simulink library "FaultInsertionUnit"  (Simulink 8.0)
settings: Solver=ode45  StartTime=0.0  StopTime=10.0  RelTol=1e-3
undefined symbols (not defined in the file): Ts
libraries: simulink x16
(part 1 of 2)
settings Model: Creator=jroth  LastModifiedBy=jroth

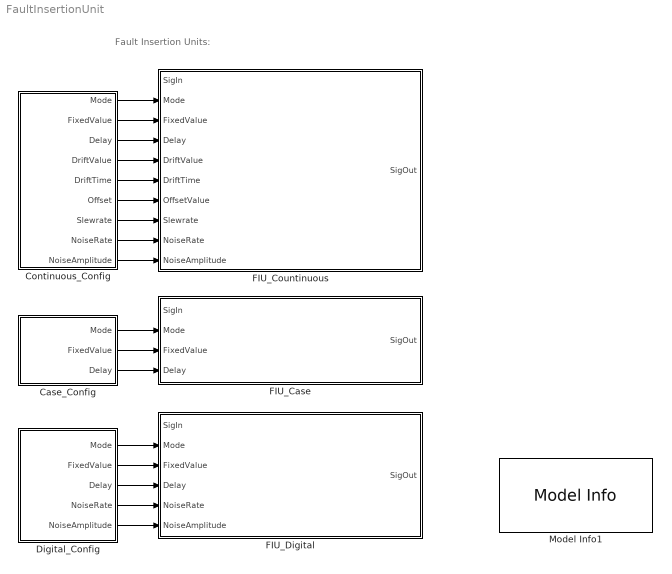
== system FaultInsertionUnit ==
  note: Fault Insertion Units:
  Case_Config : Subsystem
  Continuous_Config : Subsystem
  Digital_Config : Subsystem
  FIU_Case : Subsystem
  FIU_Countinuous : Subsystem
  FIU_Digital : Subsystem
  Model Info1 : simulink/Model-Wide Utilities/Model Info  InitialBlockCM=None  BlockCM=None  Frame=on  DisplayStringWithTags=|  HorizontalTextAlignment=Center  LeftAlignmentValue=0.5  SourceBlockDiagram=FaultInsertionUnit  TagMaxNumber=20
      | Version:
      | %<Creator>
      | %<ModifiedDate>
      | %<ModelVersion>
  wires:
  Case_Config/1(Mode) -> FIU_Case/2(Mode)
  Case_Config/2(FixedValue) -> FIU_Case/3(FixedValue)
  Case_Config/3(Delay) -> FIU_Case/4(Delay)
  Digital_Config/1(Mode) -> FIU_Digital/2(Mode)
  Digital_Config/2(FixedValue) -> FIU_Digital/3(FixedValue)
  Digital_Config/3(Delay) -> FIU_Digital/4(Delay)
  Digital_Config/4(NoiseRate) -> FIU_Digital/5(NoiseRate)
  Digital_Config/5(NoiseAmplitude) -> FIU_Digital/6(NoiseAmplitude)
  Continuous_Config/9(NoiseAmplitude) -> FIU_Countinuous/10(NoiseAmplitude)
  Continuous_Config/8(NoiseRate) -> FIU_Countinuous/9(NoiseRate)
  Continuous_Config/7(Slewrate) -> FIU_Countinuous/8(Slewrate)
  Continuous_Config/2(FixedValue) -> FIU_Countinuous/3(FixedValue)
  Continuous_Config/1(Mode) -> FIU_Countinuous/2(Mode)
  Continuous_Config/3(Delay) -> FIU_Countinuous/4(Delay)
  Continuous_Config/4(DriftValue) -> FIU_Countinuous/5(DriftValue)
  Continuous_Config/5(DriftTime) -> FIU_Countinuous/6(DriftTime)
  Continuous_Config/6(Offset) -> FIU_Countinuous/7(OffsetValue)

== system FaultInsertionUnit/Case_Config ==
  Auto Mode Selection : Subsystem
  Set Delay : Constant  Value=0
  Set FixedValue : Constant  Value=0
  Set Freeze : Constant  Value=0
  Mode : Outport
  FixedValue : Outport  Port=2
  Delay : Outport  Port=3
  wires:
  Set Delay/1 -> Delay/1, Auto Mode Selection/3(Check Delay)
  Set FixedValue/1 -> Auto Mode Selection/1(Check FixedValue), FixedValue/1
  Auto Mode Selection/1(Out1) -> Mode/1
  Set Freeze/1 -> Auto Mode Selection/2(Check Freeze)

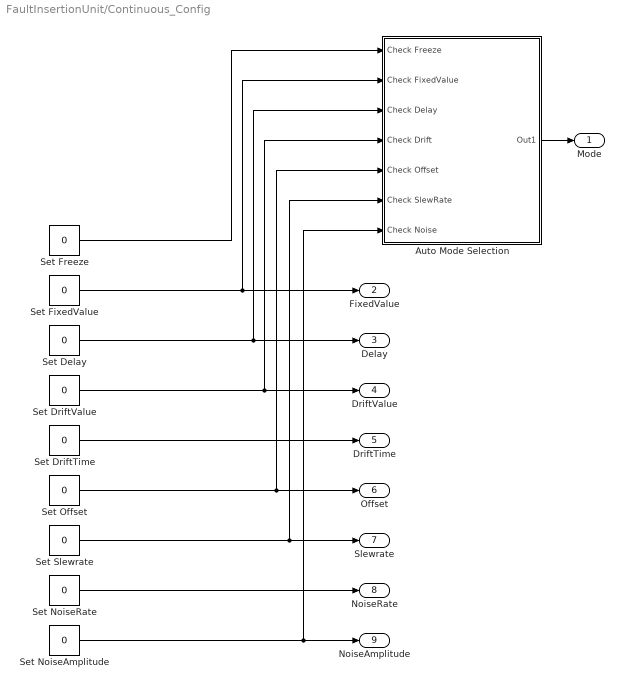
== system FaultInsertionUnit/Continuous_Config ==
  Auto Mode Selection : Subsystem
  Set Delay : Constant  Value=0
  Set DriftTime : Constant  Value=0
  Set DriftValue : Constant  Value=0
  Set FixedValue : Constant  Value=0
  Set Freeze : Constant  Value=0
  Set NoiseAmplitude : Constant  Value=0
  Set NoiseRate : Constant  Value=0
  Set Offset : Constant  Value=0
  Set Slewrate : Constant  Value=0
  Mode : Outport
  FixedValue : Outport  Port=2
  Delay : Outport  Port=3
  DriftValue : Outport  Port=4
  DriftTime : Outport  Port=5
  Offset : Outport  Port=6
  Slewrate : Outport  Port=7
  NoiseRate : Outport  Port=8
  NoiseAmplitude : Outport  Port=9
  wires:
  Set NoiseRate/1 -> NoiseRate/1
  Set Delay/1 -> Auto Mode Selection/3(Check Delay), Delay/1
  Set Offset/1 -> Auto Mode Selection/5(Check Offset), Offset/1
  Set FixedValue/1 -> Auto Mode Selection/2(Check FixedValue), FixedValue/1
  Set NoiseAmplitude/1 -> Auto Mode Selection/7(Check Noise), NoiseAmplitude/1
  Set Slewrate/1 -> Auto Mode Selection/6(Check SlewRate), Slewrate/1
  Auto Mode Selection/1(Out1) -> Mode/1
  Set DriftValue/1 -> Auto Mode Selection/4(Check Drift), DriftValue/1
  Set DriftTime/1 -> DriftTime/1
  Set Freeze/1 -> Auto Mode Selection/1(Check Freeze)

== system FaultInsertionUnit/Digital_Config ==
  Auto Mode Selection : Subsystem
  Set Delay : Constant  Value=0
  Set FixedValue : Constant  Value=0
  Set Freeze : Constant  Value=0
  Set Negate : Constant  Value=0
  Set NoiseAmplitude : Constant  Value=0
  Set NoiseRate : Constant  Value=0
  Mode : Outport
  FixedValue : Outport  Port=2
  Delay : Outport  Port=3
  NoiseRate : Outport  Port=4
  NoiseAmplitude : Outport  Port=5
  wires:
  Set NoiseRate/1 -> NoiseRate/1
  Set Delay/1 -> Auto Mode Selection/4(Check Delay), Delay/1
  Set Negate/1 -> Auto Mode Selection/2(Check Negate)
  Set FixedValue/1 -> Auto Mode Selection/1(Check FixedValue), FixedValue/1
  Set NoiseAmplitude/1 -> Auto Mode Selection/5(Check Noise), NoiseAmplitude/1
  Auto Mode Selection/1(Out1) -> Mode/1
  Set Freeze/1 -> Auto Mode Selection/3(Check Freeze)

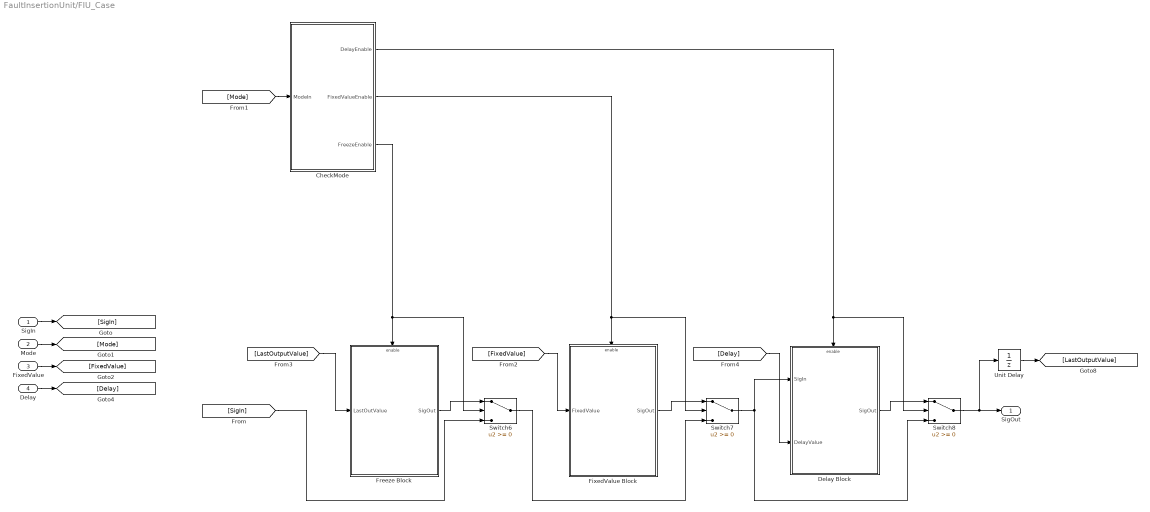
== system FaultInsertionUnit/FIU_Case ==
  SigIn : Inport
  Mode : Inport  Port=2
  FixedValue : Inport  Port=3
  Delay : Inport  Port=4
  CheckMode : Subsystem
  Delay Block : Subsystem
  FixedValue Block : Subsystem  TreatAsAtomicUnit=on
  Freeze Block : Subsystem  TreatAsAtomicUnit=on
  Switch6 : Switch
  Switch7 : Switch
  Switch8 : Switch
  Unit Delay : UnitDelay  SampleTime=-1
  SigOut : Outport
  wires:
  [FixedValue] -> FixedValue Block/1(FixedValue)
  Delay Block/1(SigOut) -> Switch8/1
  Switch7/1 -> Delay Block/1(SigIn), Switch8/3
  [Delay] -> Delay Block/2(DelayValue)
  [SigIn] -> Switch6/3
  CheckMode/3(FreezeEnable) -> Switch6/2, Freeze Block/Enable
  Switch6/1 -> Switch7/3
  CheckMode/2(FixedValueEnable) -> Switch7/2, FixedValue Block/Enable
  CheckMode/1(DelayEnable) -> Switch8/2, Delay Block/Enable
  FixedValue Block/1(SigOut) -> Switch7/1
  Freeze Block/1(SigOut) -> Switch6/1
  SigIn/1 -> [SigIn]
  Mode/1 -> [Mode]
  FixedValue/1 -> [FixedValue]
  Delay/1 -> [Delay]
  [Mode] -> CheckMode/1(ModeIn)
  Switch8/1 -> Unit Delay/1, SigOut/1
  [LastOutputValue] -> Freeze Block/1(LastOutValue)
  Unit Delay/1 -> [LastOutputValue]

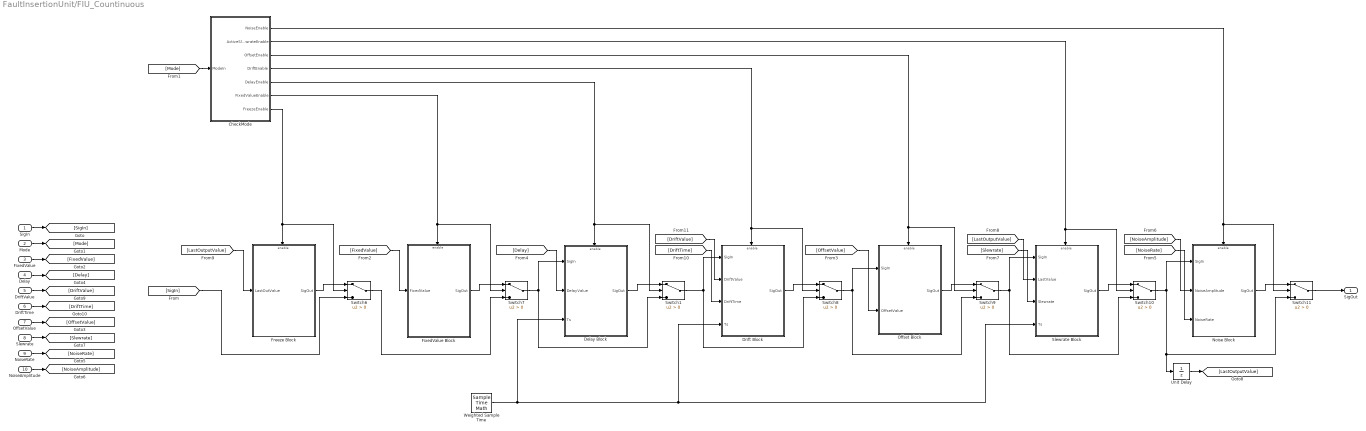
== system FaultInsertionUnit/FIU_Countinuous ==
  SigIn : Inport
  Mode : Inport  Port=2
  FixedValue : Inport  Port=3
  Delay : Inport  Port=4
  DriftValue : Inport  Port=5
  DriftTime : Inport  Port=6
  OffsetValue : Inport  Port=7
  Slewrate : Inport  Port=8
  NoiseRate : Inport  Port=9
  NoiseAmplitude : Inport  Port=10
  CheckMode : Subsystem
  Delay Block : Subsystem
  Drift Block : Subsystem  TreatAsAtomicUnit=on
  FixedValue Block : Subsystem  TreatAsAtomicUnit=on
  Freeze Block : Subsystem  TreatAsAtomicUnit=on
      mask Display: image(imread('freeze.jpg'))
  Noise Block : Subsystem
  Offset Block : Subsystem
  Slewrate Block : Subsystem
  Switch{1,6..11} (7 alike) : Switch  Criteria=u2 > Threshold
  Unit Delay : UnitDelay  SampleTime=-1
  Weighted Sample Time : SampleTimeMath  TsampMathOp=Ts Only
  SigOut : Outport
  wires:
  [FixedValue] -> FixedValue Block/1(FixedValue)
  Slewrate Block/1(SigOut) -> Switch10/1
  [Slewrate] -> Slewrate Block/3(Slewrate)
  Offset Block/1(SigOut) -> Switch9/1
  Switch9/1 -> Slewrate Block/1(SigIn), Switch10/3
  [NoiseRate] -> Noise Block/3(NoiseRate)
  Switch7/1 -> Switch1/3, Delay Block/1(SigIn)
  [NoiseAmplitude] -> Noise Block/2(NoiseAmplitude)
  Switch10/1 -> Unit Delay/1, Switch11/3, Noise Block/1(SigIn)
  [Delay] -> Delay Block/2(DelayValue)
  Noise Block/1(SigOut) -> Switch11/1
  [LastOutputValue] -> Slewrate Block/2(LastValue)
  [OffsetValue] -> Offset Block/2(OffsetValue)
  Switch8/1 -> Switch9/3, Offset Block/1(SigIn)
  [SigIn] -> Switch6/3
  CheckMode/7(FreezeEnable) -> Switch6/2, Freeze Block/Enable
  Switch6/1 -> Switch7/3
  CheckMode/6(FixedValueEnable) -> Switch7/2, FixedValue Block/Enable
  CheckMode/2(ActiveSlewrateEnable) -> Switch10/2, Slewrate Block/Enable
  CheckMode/1(NoiseEnable) -> Switch11/2, Noise Block/Enable
  FixedValue Block/1(SigOut) -> Switch7/1
  Freeze Block/1(SigOut) -> Switch6/1
  SigIn/1 -> [SigIn]
  Mode/1 -> [Mode]
  FixedValue/1 -> [FixedValue]
  OffsetValue/1 -> [OffsetValue]
  Delay/1 -> [Delay]
  NoiseRate/1 -> [NoiseRate]
  NoiseAmplitude/1 -> [NoiseAmplitude]
  Slewrate/1 -> [Slewrate]
  Unit Delay/1 -> [LastOutputValue]
  [Mode] -> CheckMode/1(ModeIn)
  Switch11/1 -> SigOut/1
  [LastOutputValue] -> Freeze Block/1(LastOutValue)
  CheckMode/3(OffsetEnable) -> Offset Block/Enable, Switch9/2
  Weighted Sample Time/1 -> Delay Block/3(Ts), Slewrate Block/4(Ts), Drift Block/4(Ts)
  CheckMode/5(DelayEnable) -> Switch1/2, Delay Block/Enable
  Switch1/1 -> Switch8/3, Drift Block/1(SigIn)
  DriftValue/1 -> [DriftValue]
  DriftTime/1 -> [DriftTime]
  Delay Block/1(SigOut) -> Switch1/1
  Drift Block/1(SigOut) -> Switch8/1
  CheckMode/4(DriftEnable) -> Switch8/2, Drift Block/Enable
  [DriftValue] -> Drift Block/2(DriftValue)
  [DriftTime] -> Drift Block/3(DriftTime)

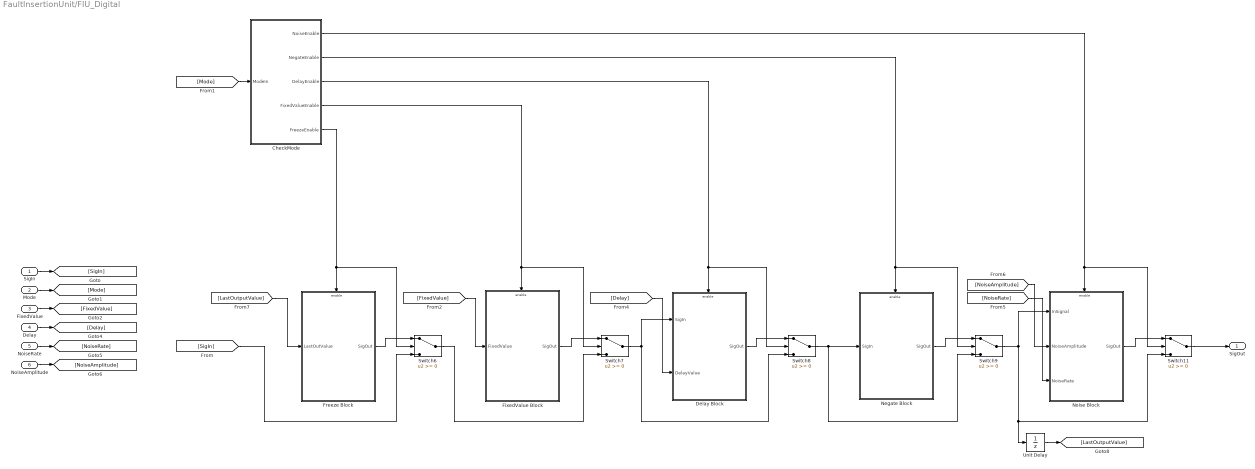
== system FaultInsertionUnit/FIU_Digital ==
  SigIn : Inport
  Mode : Inport  Port=2
  FixedValue : Inport  Port=3
  Delay : Inport  Port=4
  NoiseRate : Inport  Port=5
  NoiseAmplitude : Inport  Port=6
  CheckMode : Subsystem
  Delay Block : Subsystem
  FixedValue Block : Subsystem  TreatAsAtomicUnit=on
  Freeze Block : Subsystem  TreatAsAtomicUnit=on
  Negate Block : Subsystem
  Noise Block : Subsystem
  Switch{6..9,11} (5 alike) : Switch
  Unit Delay : UnitDelay  SampleTime=-1
  SigOut : Outport
  wires:
  [FixedValue] -> FixedValue Block/1(FixedValue)
  Negate Block/1(SigOut) -> Switch9/1
  Delay Block/1(SigOut) -> Switch8/1
  Switch7/1 -> Delay Block/1(SigIn), Switch8/3
  Switch9/1 -> Noise Block/1(InSignal), Unit Delay/1, Switch11/3
  [Delay] -> Delay Block/2(DelayValue)
  Switch8/1 -> Switch9/3, Negate Block/1(SigIn)
  [SigIn] -> Switch6/3
  CheckMode/5(FreezeEnable) -> Switch6/2, Freeze Block/Enable
  Switch6/1 -> Switch7/3
  CheckMode/4(FixedValueEnable) -> Switch7/2, FixedValue Block/Enable
  CheckMode/3(DelayEnable) -> Switch8/2, Delay Block/Enable
  CheckMode/2(NegateEnable) -> Switch9/2, Negate Block/Enable
  CheckMode/1(NoiseEnable) -> Switch11/2, Noise Block/Enable
  FixedValue Block/1(SigOut) -> Switch7/1
  Freeze Block/1(SigOut) -> Switch6/1
  SigIn/1 -> [SigIn]
  Mode/1 -> [Mode]
  FixedValue/1 -> [FixedValue]
  Delay/1 -> [Delay]
  NoiseRate/1 -> [NoiseRate]
  NoiseAmplitude/1 -> [NoiseAmplitude]
  Unit Delay/1 -> [LastOutputValue]
  [Mode] -> CheckMode/1(ModeIn)
  Switch11/1 -> SigOut/1
  [NoiseAmplitude] -> Noise Block/2(NoiseAmplitude)
  [NoiseRate] -> Noise Block/3(NoiseRate)
  Noise Block/1(SigOut) -> Switch11/1
  [LastOutputValue] -> Freeze Block/1(LastOutValue)

== system FaultInsertionUnit/Case_Config/Auto Mode Selection ==
  Check FixedValue : Inport
  Check Freeze : Inport  Port=2
  Check Delay : Inport  Port=3
  Constant : Constant  Value=2
  Constant2 : Constant
  Constant3 : Constant  Value=4
  Data Type Conversion : DataTypeConversion  OutDataTypeStr=uint8
  Sum : Sum  Inputs=|++
  Sum4 : Sum  Inputs=|++
  Switch : Switch  Criteria=u2 ~= 0
  Switch2 : Switch  Criteria=u2 ~= 0
  Switch3 : Switch  Criteria=u2 ~= 0
  Out1 : Outport
  wires:
  Constant2/1 -> Switch2/1
  Sum/1 -> Sum4/1
  Switch2/1 -> Sum/1
  Switch3/1 -> Sum/2
  Check Delay/1 -> Switch3/3, Switch3/2
  Switch/1 -> Sum4/2
  Check Freeze/1 -> Switch2/3, Switch2/2
  Check FixedValue/1 -> Switch/3, Switch/2
  Constant/1 -> Switch/1
  Constant3/1 -> Switch3/1
  Data Type Conversion/1 -> Out1/1
  Sum4/1 -> Data Type Conversion/1

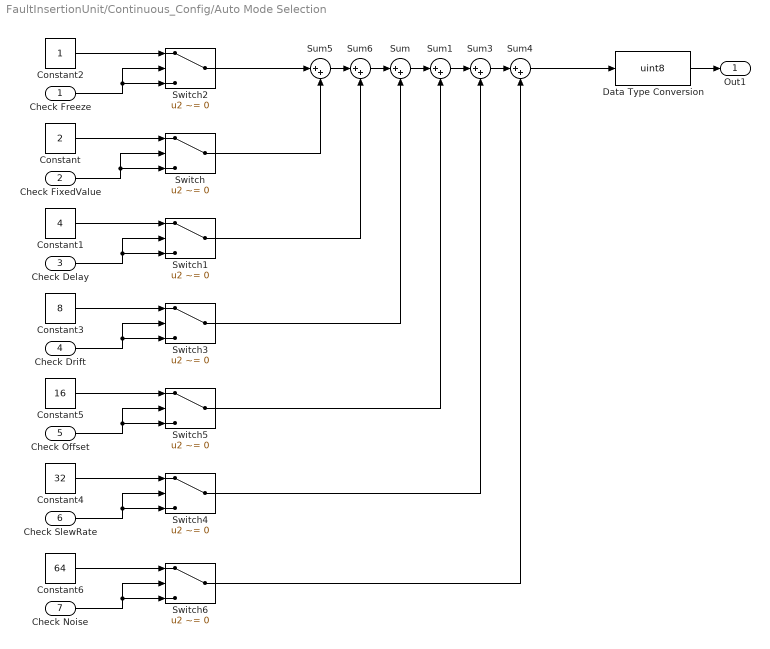
== system FaultInsertionUnit/Continuous_Config/Auto Mode Selection ==
  Check Freeze : Inport
  Check FixedValue : Inport  Port=2
  Check Delay : Inport  Port=3
  Check Drift : Inport  Port=4
  Check Offset : Inport  Port=5
  Check SlewRate : Inport  Port=6
  Check Noise : Inport  Port=7
  Constant : Constant  Value=2
  Constant1 : Constant  Value=4
  Constant2 : Constant
  Constant3 : Constant  Value=8
  Constant4 : Constant  Value=32
  Constant5 : Constant  Value=16
  Constant6 : Constant  Value=64
  Data Type Conversion : DataTypeConversion  OutDataTypeStr=uint8
  Sum{,1,3..6} (6 alike) : Sum  Inputs=|++
  Switch{,1..6} (7 alike) : Switch  Criteria=u2 ~= 0
  Out1 : Outport
  wires:
  Sum1/1 -> Sum3/1
  Constant2/1 -> Switch2/1
  Sum3/1 -> Sum4/1
  Sum/1 -> Sum1/1
  Check Drift/1 -> Switch3/3, Switch3/2
  Check Freeze/1 -> Switch2/3, Switch2/2
  Check Delay/1 -> Switch1/3, Switch1/2
  Check SlewRate/1 -> Switch4/3, Switch4/2
  Check FixedValue/1 -> Switch/3, Switch/2
  Constant/1 -> Switch/1
  Constant4/1 -> Switch4/1
  Constant1/1 -> Switch1/1
  Constant3/1 -> Switch3/1
  Data Type Conversion/1 -> Out1/1
  Check Offset/1 -> Switch5/3, Switch5/2
  Constant5/1 -> Switch5/1
  Sum4/1 -> Data Type Conversion/1
  Check Noise/1 -> Switch6/3, Switch6/2
  Constant6/1 -> Switch6/1
  Sum5/1 -> Sum6/1
  Sum6/1 -> Sum/1
  Switch2/1 -> Sum5/1
  Switch/1 -> Sum5/2
  Switch1/1 -> Sum6/2
  Switch3/1 -> Sum/2
  Switch5/1 -> Sum1/2
  Switch4/1 -> Sum3/2
  Switch6/1 -> Sum4/2

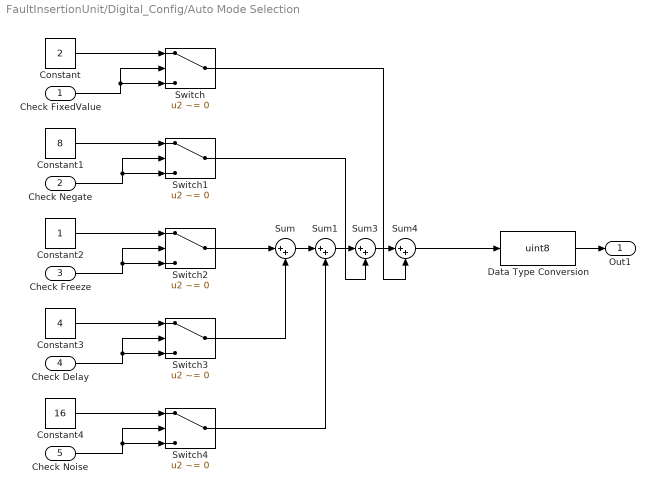
== system FaultInsertionUnit/Digital_Config/Auto Mode Selection ==
  Check FixedValue : Inport
  Check Negate : Inport  Port=2
  Check Freeze : Inport  Port=3
  Check Delay : Inport  Port=4
  Check Noise : Inport  Port=5
  Constant : Constant  Value=2
  Constant1 : Constant  Value=8
  Constant2 : Constant
  Constant3 : Constant  Value=4
  Constant4 : Constant  Value=16
  Data Type Conversion : DataTypeConversion  OutDataTypeStr=uint8
  Sum{,1,3..4} (4 alike) : Sum  Inputs=|++
  Switch{,1..4} (5 alike) : Switch  Criteria=u2 ~= 0
  Out1 : Outport
  wires:
  Sum1/1 -> Sum3/1
  Constant2/1 -> Switch2/1
  Sum3/1 -> Sum4/1
  Switch2/1 -> Sum/1
  Switch3/1 -> Sum/2
  Sum/1 -> Sum1/1
  Check Delay/1 -> Switch3/3, Switch3/2
  Switch1/1 -> Sum3/2
  Switch4/1 -> Sum1/2
  Switch/1 -> Sum4/2
  Check Freeze/1 -> Switch2/3, Switch2/2
  Check Negate/1 -> Switch1/3, Switch1/2
  Check Noise/1 -> Switch4/3, Switch4/2
  Check FixedValue/1 -> Switch/3, Switch/2
  Constant/1 -> Switch/1
  Constant4/1 -> Switch4/1
  Constant1/1 -> Switch1/1
  Constant3/1 -> Switch3/1
  Data Type Conversion/1 -> Out1/1
  Sum4/1 -> Data Type Conversion/1

== system FaultInsertionUnit/FIU_Case/CheckMode ==
  ModeIn : Inport  OutDataTypeStr=uint8
  CheckDelayEnable : simulink/Logic and Bit Operations/Bitwise Operator  logicop=AND  UseBitMask=on  BitMask=bin2dec('00000100')  BitMaskRealWorld=Stored Integer
  CheckFixedValueEnable : simulink/Logic and Bit Operations/Bitwise Operator  logicop=AND  UseBitMask=on  BitMask=bin2dec('00000010')  BitMaskRealWorld=Stored Integer
  CheckFreezeEnable : simulink/Logic and Bit Operations/Bitwise Operator  logicop=AND  UseBitMask=on  BitMask=bin2dec('00000001')  BitMaskRealWorld=Stored Integer
  Data Type Conversion : DataTypeConversion  OutDataTypeStr=boolean
  Data Type Conversion1 : DataTypeConversion  OutDataTypeStr=boolean
  Data Type Conversion2 : DataTypeConversion  OutDataTypeStr=boolean
  DelayEnable : Outport
  FixedValueEnable : Outport  Port=2
  FreezeEnable : Outport  Port=3
  wires:
  CheckDelayEnable/1 -> Data Type Conversion2/1
  CheckFixedValueEnable/1 -> Data Type Conversion1/1
  CheckFreezeEnable/1 -> Data Type Conversion/1
  ModeIn/1 -> CheckDelayEnable/1, CheckFixedValueEnable/1, CheckFreezeEnable/1
  Data Type Conversion2/1 -> DelayEnable/1
  Data Type Conversion1/1 -> FixedValueEnable/1
  Data Type Conversion/1 -> FreezeEnable/1

== system FaultInsertionUnit/FIU_Case/Delay Block ==
  note: continuously approach to set DelayValue
  note: Detect first cycle of enabled subsystem
  SigIn : Inport
  DelayValue : Inport  Port=2
  Enable : EnablePort  StatesWhenEnabling=reset
  Constant1 : Constant  Value=0
  Subsystem : Subsystem
  Switch1 : Switch  Criteria=u2 > Threshold
  Unit Delay1 : UnitDelay  InitialCondition=1  SampleTime=-1
  Variable Time Delay : VariableTransportDelay  MaximumDelay=10  MaximumPoints=6000  FixedBuffer=on  TransDelayFeedthrough=on
  SigOut : Outport
  wires:
  DelayValue/1 -> Subsystem/1(DelayValueSet)
  Subsystem/1(DelayValueIs) -> Variable Time Delay/2
  Variable Time Delay/1 -> Switch1/3
  Switch1/1 -> SigOut/1
  Unit Delay1/1 -> Switch1/2  "EnableFirstCycle"
  Constant1/1 -> Unit Delay1/1
  SigIn/1 -> Switch1/1, Variable Time Delay/1

== system FaultInsertionUnit/FIU_Case/FixedValue Block ==
  FixedValue : Inport
  Enable : EnablePort
  SigOut : Outport
  wires:
  FixedValue/1 -> SigOut/1

== system FaultInsertionUnit/FIU_Case/Freeze Block ==
  LastOutValue : Inport
  Enable : EnablePort
  SigOut : Outport
  wires:
  LastOutValue/1 -> SigOut/1

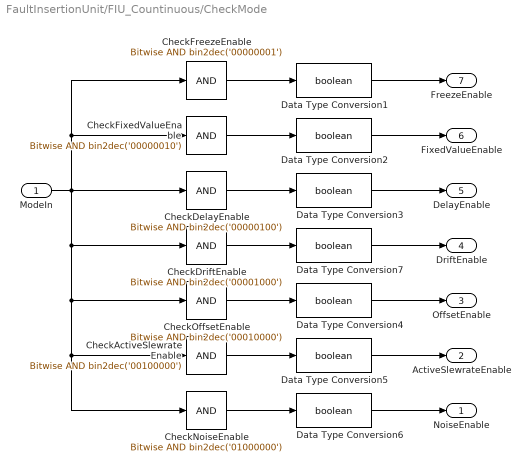
== system FaultInsertionUnit/FIU_Countinuous/CheckMode ==
  ModeIn : Inport  OutDataTypeStr=uint8
  CheckActiveSlewrateEnable : simulink/Logic and Bit Operations/Bitwise Operator  logicop=AND  UseBitMask=on  BitMask=bin2dec('00100000')  BitMaskRealWorld=Stored Integer
  CheckDelayEnable : simulink/Logic and Bit Operations/Bitwise Operator  logicop=AND  UseBitMask=on  BitMask=bin2dec('00000100')  BitMaskRealWorld=Stored Integer
  CheckDriftEnable : simulink/Logic and Bit Operations/Bitwise Operator  logicop=AND  UseBitMask=on  BitMask=bin2dec('00001000')  BitMaskRealWorld=Stored Integer
  CheckFixedValueEnable : simulink/Logic and Bit Operations/Bitwise Operator  logicop=AND  UseBitMask=on  BitMask=bin2dec('00000010')  BitMaskRealWorld=Stored Integer
  CheckFreezeEnable : simulink/Logic and Bit Operations/Bitwise Operator  logicop=AND  UseBitMask=on  BitMask=bin2dec('00000001')  BitMaskRealWorld=Stored Integer
  CheckNoiseEnable : simulink/Logic and Bit Operations/Bitwise Operator  logicop=AND  UseBitMask=on  BitMask=bin2dec('01000000')  BitMaskRealWorld=Stored Integer
  CheckOffsetEnable : simulink/Logic and Bit Operations/Bitwise Operator  logicop=AND  UseBitMask=on  BitMask=bin2dec('00010000')  BitMaskRealWorld=Stored Integer
  Data Type Conversion{1..7} (7 alike) : DataTypeConversion  OutDataTypeStr=boolean
  NoiseEnable : Outport
  ActiveSlewrateEnable : Outport  Port=2
  OffsetEnable : Outport  Port=3
  DriftEnable : Outport  Port=4
  DelayEnable : Outport  Port=5
  FixedValueEnable : Outport  Port=6
  FreezeEnable : Outport  Port=7
  wires:
  CheckNoiseEnable/1 -> Data Type Conversion6/1
  CheckActiveSlewrateEnable/1 -> Data Type Conversion5/1
  CheckFixedValueEnable/1 -> Data Type Conversion2/1
  CheckFreezeEnable/1 -> Data Type Conversion1/1
  Data Type Conversion6/1 -> NoiseEnable/1
  Data Type Conversion5/1 -> ActiveSlewrateEnable/1
  Data Type Conversion2/1 -> FixedValueEnable/1
  Data Type Conversion1/1 -> FreezeEnable/1
  CheckDelayEnable/1 -> Data Type Conversion3/1
  CheckOffsetEnable/1 -> Data Type Conversion4/1
  Data Type Conversion4/1 -> OffsetEnable/1
  Data Type Conversion3/1 -> DelayEnable/1
  CheckDriftEnable/1 -> Data Type Conversion7/1
  ModeIn/1 -> CheckDriftEnable/1, CheckNoiseEnable/1, CheckActiveSlewrateEnable/1, CheckOffsetEnable/1, CheckDelayEnable/1, CheckFixedValueEnable/1, CheckFreezeEnable/1
  Data Type Conversion7/1 -> DriftEnable/1

== system FaultInsertionUnit/FIU_Countinuous/Delay Block ==
  note: Detect first cycle of enabled subsystem
  SigIn : Inport
  DelayValue : Inport  Port=2
  Ts : Inport  Port=3
  Enable : EnablePort  StatesWhenEnabling=reset
  Constant1 : Constant  Value=0
  Divide : Product  Inputs=*/
  Subsystem : Subsystem
  Switch1 : Switch  Criteria=u2 > Threshold
  Unit Delay1 : UnitDelay  InitialCondition=1  SampleTime=-1
  Variable Integer Delay (max. 10 seconds) : Delay  DelayLengthSource=Input port  DelayLengthUpperLimit=10000
      settings: InputPortMap=u0,p1
  SigOut : Outport
  wires:
  Variable Integer Delay (max. 10 seconds)/1 -> Switch1/3
  Switch1/1 -> SigOut/1
  Unit Delay1/1 -> Switch1/2  "EnableFirstCycle"
  Constant1/1 -> Unit Delay1/1
  SigIn/1 -> Variable Integer Delay (max. 10 seconds)/1, Switch1/1
  DelayValue/1 -> Divide/1
  Ts/1 -> Divide/2
  Divide/1 -> Variable Integer Delay (max. 10 seconds)/2

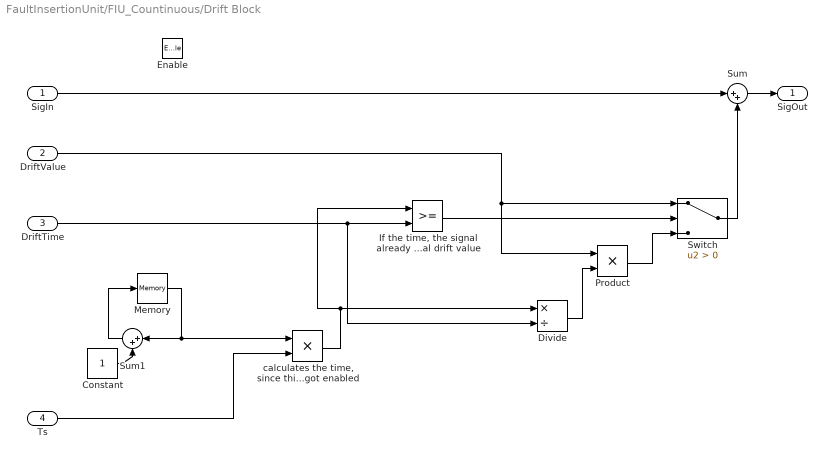
== system FaultInsertionUnit/FIU_Countinuous/Drift Block ==
  SigIn : Inport
  DriftValue : Inport  Port=2
  DriftTime : Inport  Port=3
  Ts : Inport  Port=4
  Enable : EnablePort
  Constant : Constant
  Divide : Product  Inputs=*/
  "If the time, the signal already drifted is greater than the drift time, just add an offset else add the proportional drift value" : RelationalOperator  OutDataTypeStr=boolean
  Memory : Memory
  Product : Product  RndMeth=Zero
  Sum : Sum  Inputs=|++
  Sum1 : Sum  Inputs=|++
  Switch : Switch  Criteria=u2 > Threshold
  "calculates the time, since this block got enabled" : Product  RndMeth=Zero
  SigOut : Outport
  wires:
  Sum/1 -> SigOut/1
  SigIn/1 -> Sum/1
  DriftValue/1 -> Product/1, Switch/1
  Switch/1 -> Sum/2
  Memory/1 -> "calculates the time, since this block got enabled"/1, Sum1/1
  Sum1/1 -> Memory/1
  Constant/1 -> Sum1/2
  Ts/1 -> "calculates the time, since this block got enabled"/2
  "calculates the time, since this block got enabled"/1 -> Divide/1, "If the time, the signal already drifted is greater than the drift time, just add an offset else add the proportional drift value"/1
  "If the time, the signal already drifted is greater than the drift time, just add an offset else add the proportional drift value"/1 -> Switch/2
  DriftTime/1 -> "If the time, the signal already drifted is greater than the drift time, just add an offset else add the proportional drift value"/2, Divide/2
  Product/1 -> Switch/3
  Divide/1 -> Product/2

== system FaultInsertionUnit/FIU_Countinuous/FixedValue Block ==
  FixedValue : Inport
  Enable : EnablePort
  SigOut : Outport
  wires:
  FixedValue/1 -> SigOut/1

== system FaultInsertionUnit/FIU_Countinuous/Freeze Block ==
  LastOutValue : Inport
  Enable : EnablePort
  SigOut : Outport
  wires:
  LastOutValue/1 -> SigOut/1

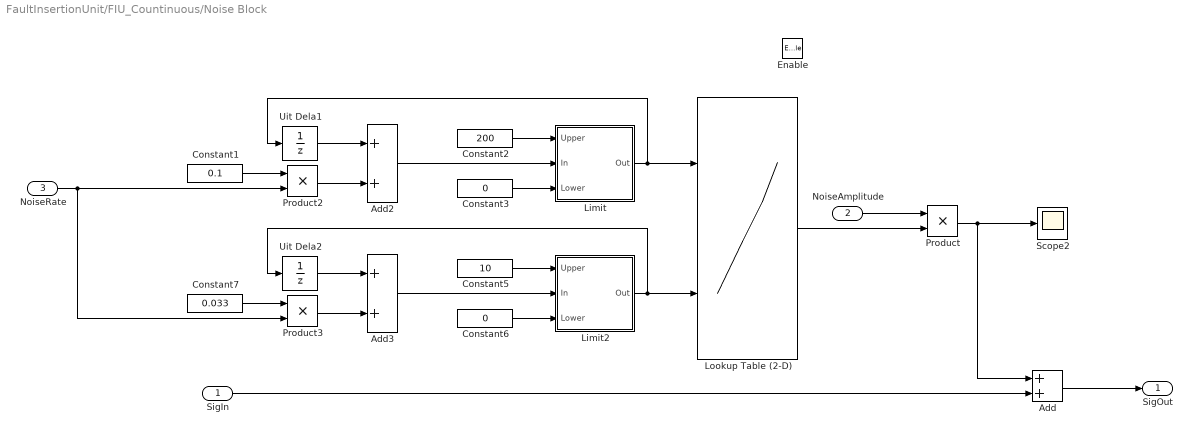
== system FaultInsertionUnit/FIU_Countinuous/Noise Block ==
  SigIn : Inport
  NoiseAmplitude : Inport  Port=2  OutDataTypeStr=double
  NoiseRate : Inport  Port=3
  Enable : EnablePort  StatesWhenEnabling=reset
  Add : Sum
  Add2 : Sum
  Add3 : Sum
  Constant1 : Constant  Value=0.1
  Constant2 : Constant  Value=200
  Constant3 : Constant  Value=0
  Constant5 : Constant  Value=10
  Constant6 : Constant  Value=0
  Constant7 : Constant  Value=0.033
  Limit : Subsystem
  Limit2 : Subsystem
  Lookup Table (2-D) : Lookup2D  RowIndex=[1:200]  ColumnIndex=[1:10]  Table=[0.059478 0.43661 -0.49306 0.23102 0.047775 0.32881 0.10527 -0.96761 -0.17936 -0.7715 ;-0.46458 -0.14226 -0.073569 -0.13391 -0.068713 -0.51372 -0.048223 -0.05778 -0.033297 -0.9336 ;0.69392 -0.63036 -0.42447 0.87456 0.21707 -0.02388 -0.10525 0.04543 0.19352 0.95965 ;-0.57043 -0.68679 0.90023 0.18436 0.88412 0.36409 -0.60649 0.27584 -0.46311 0.076011 ;0.51483 0.44455 -0.31639 0.44814 -0.79573 -0.91568 0.69359 0.52856 -0.51749 -0.27781 ;-0.46372 -0.7295 -0.58356 0.46135 0.76716 0.6258 -0.61754 0.45535 -0.73541 -0.86835 ;0.50488 0.74498 -0.20318 -0.26701 -0.2636 0.17345 0.55475 0.47207 -0.91499 -0.097736 ;-0.64441 -0.89804 0.34354 0.37527 0.28775 -0.9859 0.6495 -0.15923 0.78148 -0.35851 ;0.76434 -0.74859 -0.95771 -0.15581 0.81145 0.077942 -0.89502 -0.80833 -0.73444 -0.05261 ;-0.24648 -0.82401 -0.55611 0.8206 -0.20482 -0.47114 -0.56003 -0.71421 -0.43614 -0.6372 ;0.9408 0.91361 -0.0079724 -0.48861 0.19346 -0.086788 -0.76528 0.52495 -0.60627 0.0036683 ;0.47479 0.24439 0.82936 0.12246 -0.34564 0.88177 -0.29726 0.39259 -0.86418 0.6683 ;-0.010681 -0.4077 -0.080105 0.38061 0.47611 -0.82642 -0.39268 -0.039043 -0.086685 0.76899 ;0.65553 0.95958 -0.96498 -0.46645 -0.84307 0.9534 0.055539 0.30511 0.052539 0.57284 ;0.089641 0.83536 0.79567 -0.23709 -0.33065 0.29781 0.18052 -0.19083 0.37514 -0.0042971 ;-0.22126 0.58358 0.14929 0.12056 0.49933 -0.094293 0.65897 -0.58568 0.95792 0.80524 ;0.99764 -0.47973 -0.52224 0.74083 0.54483 -0.86987 0.16101 0.64042 0.6324 0.42208 ;0.33707 -0.4082 -0.75139 0.60465 -0.63416 0.39138 -0.21017 0.96892 -0.70009 -0.25507 ;0.0069244 -0.39533 -0.23039 -0.65718 -0.0096847 0.7163 0.51323 -0.43487 -0.26948 -0.85631 ;0.14176 0.85986 -0.44225 0.34414 0.44564 -0.13564 -0.93444 -0.38616 -0.28968 0.88197 ;-0.89037 -0.68029 0.6924 -0.63973 0.62656 -0.67392 -0.63956 -0.67534 0.76093 -0.96337 ;0.84891 -0.35158 -0.78584 -0.51018 -0.88655 -0.56286 0.89732 0.19436 0.53456 -0.10364 ;-0.90548 0.017171 0.71119 0.60675 -0.56683 -0.2331 -0.38058 0.44347 -0.33375 0.78087 ;0.5372 0.57766 0.21542 -0.048727 0.63165 0.41196 0.91552 -0.24646 -0.25985 0.1879 ;-0.64541 -0.89197 0.75662 0.92675 0.65934 0.10358 -0.67716 0.53513 -0.31431 -0.63993 ;0.64027 -0.45024 0.29231 0.19304 -0.94798 -0.07999 -0.31727 0.60419 -0.8408 0.62697 ;-0.60565 -0.3892 -0.11436 -0.69293 0.12092 0.9043 0.61038 0.51203 -0.45509 -0.68316 ;-0.18204 0.23803 -0.41733 0.89078 -0.7563 -0.42155 0.72326 -0.6621 -0.75891 0.63369 ;-0.43066 -0.78703 0.58854 -0.72774 -0.00028933 0.85117 0.6476 0.54839 -0.6327 0.37228 ;-0.52944 -0.63109 0.38573 -0.50185 0.44127 -0.27515 0.984 -0.47949 -0.34999 -0.25508 ;0.65462 -0.57956 0.64436 -0.55375 -0.0052001 0.56542 -0.49842 -0.39404 0.90475 -0.74693 ;-0.50147 0.63867 0.68479 -0.78925 -0.037871 -0.012363 -0.13535 0.86843 -0.92309 -0.35309 ;0.63539 0.75297 -0.066481 -0.39864 -0.77222 0.81742 0.84727 0.65968 -0.11524 0.69016 ;0.46389 0.74483 0.64082 0.70691 0.038276 0.44384 0.27706 -0.24474 0.79914 0.55669 ;0.34935 0.19564 -0.72728 0.34681 -0.0074384 -0.11379 -0.27504 -0.13171 0.60629 -0.46375 ;0.63704 -0.00029838 0.59022 -0.656 0.42108 0.6068 0.91679 -0.36743 -0.67755 0.45638 ;0.073564 0.5302 0.26019 0.53598 -0.63809 -0.36186 -0.76003 0.36121 -0.99579 0.2988 ;-0.65918 0.8818 -0.64919 -0.77877 -0.81473 -0.66233 -0.35199 0.54211 0.7532 0.21177 ;-0.30082 0.77817 0.27137 -0.59429 -0.80614 -0.5918 -0.53632 0.66567 -0.46164 -0.71729 ;-0.81883 -0.72359 -0.62828 -0.9465 -0.406 -0.17584 0.23429 0.86747 0.58099 -0.96536 ;0.54349 -0.31806 0.68759 0.35242 -0.1096 0.034494 0.62059 -0.86088 -0.51413 0.6079 ;-0.10989 -0.5256 -0.84164 0.4136 -0.93726 0.69895 -0.22816 -0.85528 0.058181 0.63288 ;-0.59386 -0.28897 0.55798 0.3372 0.43239 0.70489 0.12355 -0.5017 -0.41183 -0.31337 ;-0.028857 -0.43394 0.59069 0.35613 0.12777 -0.26627 0.63609 0.56775 0.13261 0.74048 ;0.28837 0.20258 -0.12991 0.4687 0.30789 0.90887 -0.15657 0.76172 -0.25952 0.39273 ;-0.66931 -0.59911 -0.077129 0.7496 -0.3623 0.99325 -0.64122 0.81862 -0.18906 0.10203 ;-0.94851 0.25736 0.79573 -0.96018 ...(+13218 chars) ]  OutDataTypeStr=double
  Product : Product  RndMeth=Zero
  Product2 : Product  RndMeth=Zero
  Product3 : Product  RndMeth=Zero
  Scope2 : Scope
      settings: SaveName=ScopeData5
  Uit Dela1 : UnitDelay  SampleTime=-1
  Uit Dela2 : UnitDelay  SampleTime=-1
  SigOut : Outport
  wires:
  Constant7/1 -> Product3/1
  Product3/1 -> Add3/2
  NoiseRate/1 -> Product3/2, Product2/2
  Constant1/1 -> Product2/1
  Product2/1 -> Add2/2
  Constant6/1 -> Limit2/3(Lower)
  Constant5/1 -> Limit2/1(Upper)
  Limit2/1(Out) -> Lookup Table (2-D)/2, Uit Dela2/1
  Add3/1 -> Limit2/2(In)
  Uit Dela2/1 -> Add3/1
  Constant3/1 -> Limit/3(Lower)
  Constant2/1 -> Limit/1(Upper)
  Limit/1(Out) -> Lookup Table (2-D)/1, Uit Dela1/1
  Add2/1 -> Limit/2(In)
  Uit Dela1/1 -> Add2/1
  SigIn/1 -> Add/2
  Product/1 -> Scope2/1, Add/1
  Add/1 -> SigOut/1
  NoiseAmplitude/1 -> Product/1
  Lookup Table (2-D)/1 -> Product/2

== system FaultInsertionUnit/FIU_Countinuous/Offset Block ==
  SigIn : Inport
  OffsetValue : Inport  Port=2
  Enable : EnablePort
  Add : Sum
  SigOut : Outport
  wires:
  Add/1 -> SigOut/1
  OffsetValue/1 -> Add/2
  SigIn/1 -> Add/1

== system FaultInsertionUnit/FIU_Countinuous/Slewrate Block ==
  SigIn : Inport
  LastValue : Inport  Port=2
  Slewrate : Inport  Port=3
  Ts : Inport  Port=4
  Enable : EnablePort
  Add1 : Sum
  ArbitrateSignalChange : Subsystem
  Subtract1 : Sum  Inputs=+-
  SigOut : Outport
  wires:
  Ts/1 -> ArbitrateSignalChange/3(SamplingTime)
  Slewrate/1 -> ArbitrateSignalChange/2(SlewRate)
  Subtract1/1 -> ArbitrateSignalChange/1(RequestedSignalChange)
  SigIn/1 -> Subtract1/1
  Add1/1 -> SigOut/1
  LastValue/1 -> Subtract1/2, Add1/2
  ArbitrateSignalChange/1(AcceptedSignalChange) -> Add1/1

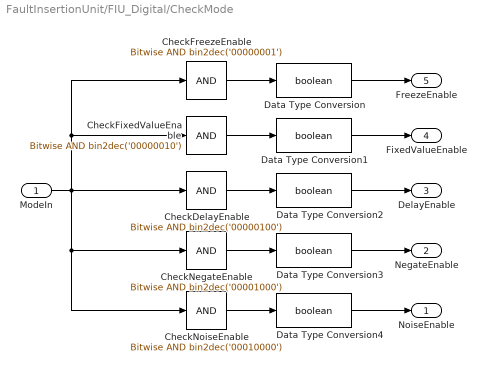
== system FaultInsertionUnit/FIU_Digital/CheckMode ==
  ModeIn : Inport  OutDataTypeStr=uint8
  CheckDelayEnable : simulink/Logic and Bit Operations/Bitwise Operator  logicop=AND  UseBitMask=on  BitMask=bin2dec('00000100')  BitMaskRealWorld=Stored Integer
  CheckFixedValueEnable : simulink/Logic and Bit Operations/Bitwise Operator  logicop=AND  UseBitMask=on  BitMask=bin2dec('00000010')  BitMaskRealWorld=Stored Integer
  CheckFreezeEnable : simulink/Logic and Bit Operations/Bitwise Operator  logicop=AND  UseBitMask=on  BitMask=bin2dec('00000001')  BitMaskRealWorld=Stored Integer
  CheckNegateEnable : simulink/Logic and Bit Operations/Bitwise Operator  logicop=AND  UseBitMask=on  BitMask=bin2dec('00001000')  BitMaskRealWorld=Stored Integer
  CheckNoiseEnable : simulink/Logic and Bit Operations/Bitwise Operator  logicop=AND  UseBitMask=on  BitMask=bin2dec('00010000')  BitMaskRealWorld=Stored Integer
  Data Type Conversion{,1..4} (5 alike) : DataTypeConversion  OutDataTypeStr=boolean
  NoiseEnable : Outport
  NegateEnable : Outport  Port=2
  DelayEnable : Outport  Port=3
  FixedValueEnable : Outport  Port=4
  FreezeEnable : Outport  Port=5
  wires:
  CheckNoiseEnable/1 -> Data Type Conversion4/1
  CheckNegateEnable/1 -> Data Type Conversion3/1
  CheckDelayEnable/1 -> Data Type Conversion2/1
  CheckFixedValueEnable/1 -> Data Type Conversion1/1
  CheckFreezeEnable/1 -> Data Type Conversion/1
  ModeIn/1 -> CheckDelayEnable/1, CheckFixedValueEnable/1, CheckFreezeEnable/1, CheckNoiseEnable/1, CheckNegateEnable/1
  Data Type Conversion/1 -> FreezeEnable/1
  Data Type Conversion1/1 -> FixedValueEnable/1
  Data Type Conversion4/1 -> NoiseEnable/1
  Data Type Conversion3/1 -> NegateEnable/1
  Data Type Conversion2/1 -> DelayEnable/1

== system FaultInsertionUnit/FIU_Digital/Delay Block ==
  note: continuously approach to set DelayValue
  note: Detect first cycle of enabled subsystem
  SigIn : Inport
  DelayValue : Inport  Port=2
  Enable : EnablePort  StatesWhenEnabling=reset
  Constant1 : Constant  Value=0
  Subsystem : Subsystem
  Switch1 : Switch  Criteria=u2 > Threshold
  Unit Delay1 : UnitDelay  InitialCondition=1  SampleTime=-1
  Variable Time Delay : VariableTransportDelay  MaximumDelay=10  MaximumPoints=6000  FixedBuffer=on  TransDelayFeedthrough=on
  SigOut : Outport
  wires:
  DelayValue/1 -> Subsystem/1(DelayValueSet)
  Subsystem/1(DelayValueIs) -> Variable Time Delay/2
  Variable Time Delay/1 -> Switch1/3
  Switch1/1 -> SigOut/1
  Unit Delay1/1 -> Switch1/2  "EnableFirstCycle"
  Constant1/1 -> Unit Delay1/1
  SigIn/1 -> Switch1/1, Variable Time Delay/1

== system FaultInsertionUnit/FIU_Digital/FixedValue Block ==
  FixedValue : Inport
  Enable : EnablePort
  SigOut : Outport
  wires:
  FixedValue/1 -> SigOut/1

== system FaultInsertionUnit/FIU_Digital/Freeze Block ==
  LastOutValue : Inport
  Enable : EnablePort
  SigOut : Outport
  wires:
  LastOutValue/1 -> SigOut/1

== system FaultInsertionUnit/FIU_Digital/Negate Block ==
  SigIn : Inport
  Enable : EnablePort
  Logical Operator : Logic  Operator=NOT  AllPortsSameDT=off  OutDataTypeStr=boolean
  SigOut : Outport
  wires:
  Logical Operator/1 -> SigOut/1
  SigIn/1 -> Logical Operator/1
